simulink model "rlChamberEnv"  (R2023b)
settings: Solver=ode45  StartTime=0.0  StopTime=3600  FixedStep=1  RelTol=1e-3
values from neighbouring files (symbols this model uses):
  Ts = 0.25    [train_agent.m]
undefined symbols (not defined in the file or in its folder): DiscIntNeverNeededParam
libraries: simulink x2, rllib x1
settings Model: Creator=hdt  LastModifiedBy=hdt
settings SolverCC: AutoInsertRateTranBlk=on

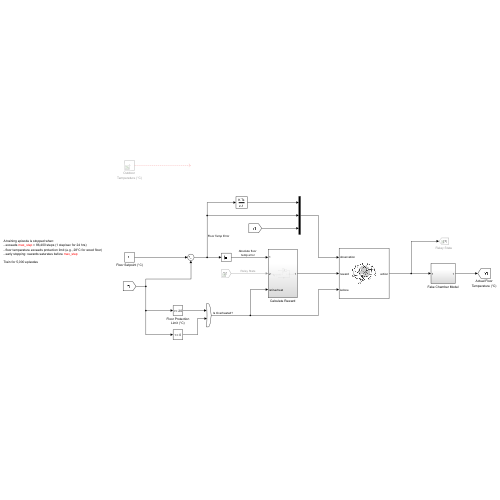
[thumbnail: Simulink's stored preview of the top-level diagram]
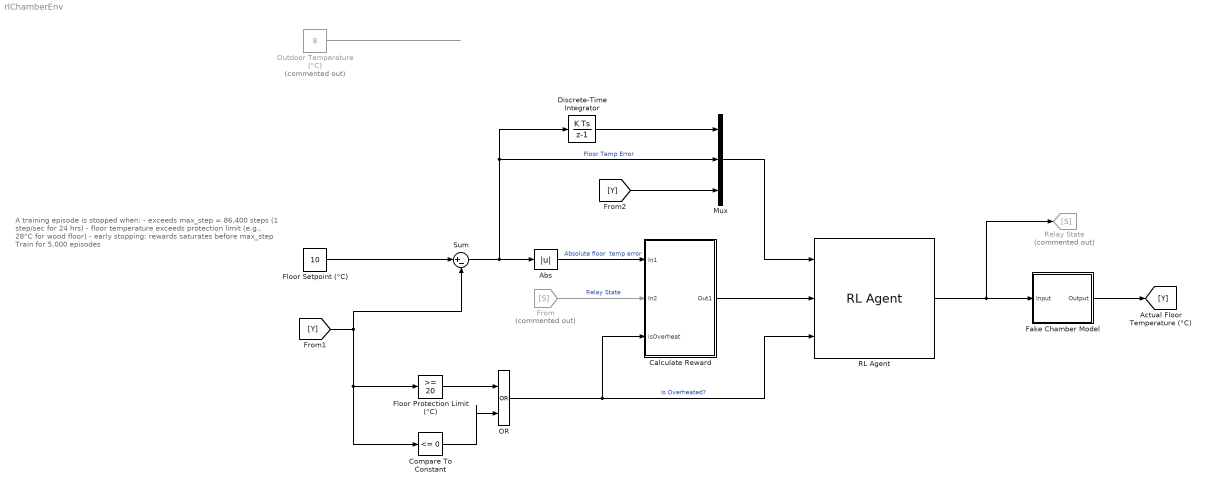
== system rlChamberEnv ==
  note: A training episode is stopped when:
      | - exceeds max_step = 86,400 steps (1 step/sec for 24 hrs)
      | - floor temperature exceeds protection limit (e.g., 28°C for wood floor)
      | - early stopping: rewards saturates before max_step
      |
      | Train for 5,000 episodes
  Abs : Abs  SaturateOnIntegerOverflow=off
  Calculate Reward : Subsystem
  Compare To Constant : simulink/Logic and Bit Operations/Compare To Constant  relop=<=  const=0  OutDataTypeStr=boolean
  Discrete-Time Integrator : DiscreteIntegrator  SampleTime=Ts  ICPrevOutput=DiscIntNeverNeededParam  ICPrevScaledInput=DiscIntNeverNeededParam
  Fake Chamber Model : Subsystem
  Floor Protection Limit (°C) : simulink/Logic and Bit Operations/Compare To Constant  relop=>=  const=20  OutDataTypeStr=boolean
  Floor Setpoint (°C) : Constant  Value=10
  From : From  Commented=on  GotoTag=S
  Mux : Mux  Inputs=3
  OR : Logic  Operator=OR  IconShape=distinctive  AllPortsSameDT=off  OutDataTypeStr=boolean
  Outdoor Temperature (°C) : Constant  Commented=on  Value=8
  RL Agent : rllib/RL Agent  Agent=agent  ExternalActionAsInput=off  ProvideLastAction=off  ProvideCumRwd=off  TreatAsDirectFeedthrough=on  UseStrictObservationDataTypes=off
  Relay State : Goto  Commented=on  GotoTag=S
  Sum : Sum  Inputs=|+-
  wires:
  Floor Setpoint (°C)/1 -> Sum/1
  Calculate Reward/1(Out1) -> RL Agent/2
  Outdoor Temperature (°C)/1 -> ?
  From/1 -> Calculate Reward/2(In2)  "Relay State"
  OR/1 -> RL Agent/3, Calculate Reward/3(isOverheat)  "Is Overheated?"
  Fake Chamber Model/1(Output) -> [Y]
  [Y] -> Compare To Constant/1, Floor Protection Limit (°C)/1, Sum/2
  Abs/1 -> Calculate Reward/1(In1)  "Absolute floor  temp error"
  RL Agent/1 -> Fake Chamber Model/1(Input), Relay State/1
  Mux/1 -> RL Agent/1
  Sum/1 -> Mux/2, Discrete-Time Integrator/1, Abs/1  "Floor Temp Error"
  Discrete-Time Integrator/1 -> Mux/1
  Floor Protection Limit (°C)/1 -> OR/1
  Compare To Constant/1 -> OR/2
  [Y] -> Mux/3

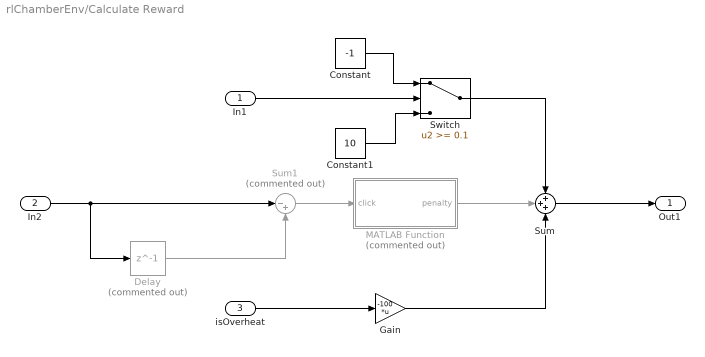
== system rlChamberEnv/Calculate Reward ==
  In1 : Inport
  In2 : Inport  Port=2
  isOverheat : Inport  Port=3
  Constant : Constant  Value=-1
  Constant1 : Constant  Value=10
  Delay : Delay  Commented=on  DelayLength=1  SampleTime=1
  Gain : Gain  Gain=-100  Multiplication=Matrix(K*u)
  MATLAB Function : MATLAB Function  Commented=on  TreatAsAtomicUnit=on
  Sum : Sum  Inputs=+++
  Sum1 : Sum  Commented=on  Inputs=|-+
  Switch : Switch  Threshold=0.1  RndMeth=Ceiling  SaturateOnIntegerOverflow=off  InputSameDT=off
  Out1 : Outport
  wires:
  In1/1 -> Switch/2
  Constant/1 -> Switch/1
  Constant1/1 -> Switch/3
  Switch/1 -> Sum/1
  In2/1 -> Sum1/1, Delay/1
  Delay/1 -> Sum1/2
  Sum1/1 -> MATLAB Function/1(click)
  MATLAB Function/1(penalty) -> Sum/2
  isOverheat/1 -> Gain/1
  Gain/1 -> Sum/3
  Sum/1 -> Out1/1

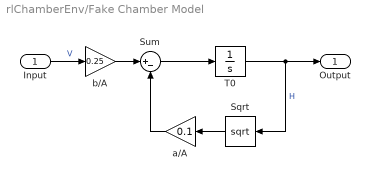
== system rlChamberEnv/Fake Chamber Model ==
  Input : Inport
  Sqrt : Sqrt  OutputSignalType=real
  Sum : Sum  Inputs=|+-  SaturateOnIntegerOverflow=on
  T0 : Integrator  InitialCondition=9.0231  LimitOutput=on  LowerSaturationLimit=0
  a/A : Gain  Gain=0.1  SaturateOnIntegerOverflow=on  OutDataTypeStr=Inherit: Same as input  ParamDataTypeStr=Inherit: Same as input
  b/A : Gain  Gain=0.25  SaturateOnIntegerOverflow=on  OutDataTypeStr=Inherit: Same as input  ParamDataTypeStr=Inherit: Same as input
  Output : Outport  VectorParamsAs1DForOutWhenUnconnected=off
  wires:
  b/A/1 -> Sum/1
  Sum/1 -> T0/1
  T0/1 -> Sqrt/1, Output/1  "H"
  Sqrt/1 -> a/A/1
  a/A/1 -> Sum/2
  Input/1 -> b/A/1  "V"

== matlab function rlChamberEnv/Calculate Reward/MATLAB Function ==
  data: click input; penalty output
function penalty = fcn(click)
    if click == 0
        penalty = 2; % No reward for every second remains unswitched
    else
        penalty = 100;
    end
end
